simulink model "COM_sl"  (R2016a)
settings: Solver=FixedStepDiscrete  StartTime=0.0  StopTime=10.0  RelTol=1e-3
undefined symbols (not defined in the file): dt
Description:
  | Template model
settings Model: ModelType=Feature  MBDTemplateVer=1.1  LastModifiedBy=jliu29
settings DataIOCC: LimitDataPoints=on
settings DebuggingCC: AllowSymbolicDim=off
settings ModelReferenceCC: PropagateSignalLabelsOutOfModel=off
settings RTWCC: Description=Generic Real-Time Target
settings GRTTargetCC: GeneratePreprocessorConditionals=Use local settings
settings ConfigComp: DVMode=PropertyProving  DVTestSuiteOptimization=CombinedObjectives (Nonlinear Extended)  DVAssertions=EnableAll  DVProofAssumptions=EnableAll  DVDisplayReport=off

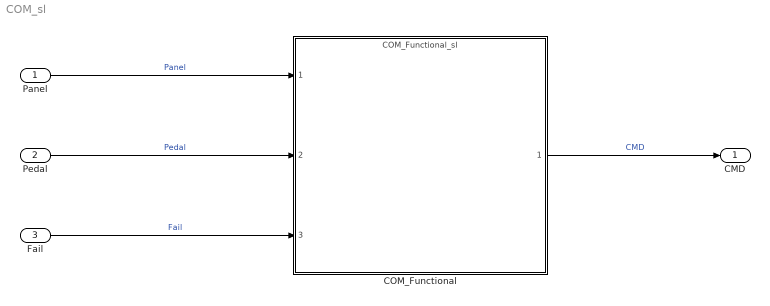
== system COM_sl ==
  Panel : Inport  OutDataTypeStr=Bus: PanelMsgImpl  SampleTime=dt  Interpolate=off  BusOutputAsStruct=on
  Pedal : Inport  Port=2  OutDataTypeStr=int32  SampleTime=dt  Interpolate=off
  Fail : Inport  Port=3  OutDataTypeStr=boolean  SampleTime=dt  Interpolate=off
  COM_Functional : ModelReference  ModelNameDialog=COM_Functional_sl.slx  SimulationMode=Normal  ModelReferenceVersion=1.2
  CMD : Outport  OutDataTypeStr=int32
  wires:
  COM_Functional/1 -> CMD/1  "CMD"
  Panel/1 -> COM_Functional/1  "Panel"
  Pedal/1 -> COM_Functional/2  "Pedal"
  Fail/1 -> COM_Functional/3  "Fail"
